simulink model "plant"  (R2026a)
settings: Solver=VariableStepAuto
undefined symbols (not defined in the file): pmsm
libraries: mcbplantlib x1, autolibpmsminterior x1
settings Model: Creator=probst  LastModifiedBy=probst

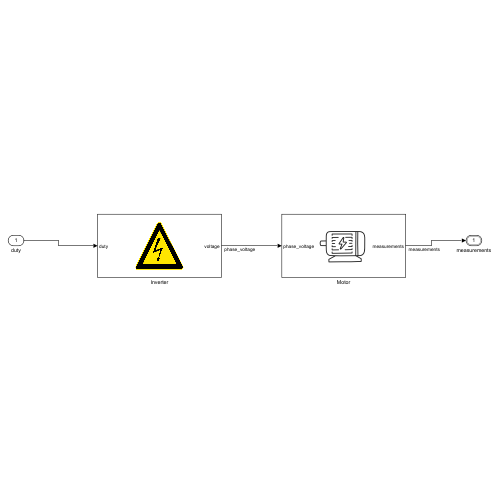
[thumbnail: Simulink's stored preview of the top-level diagram]
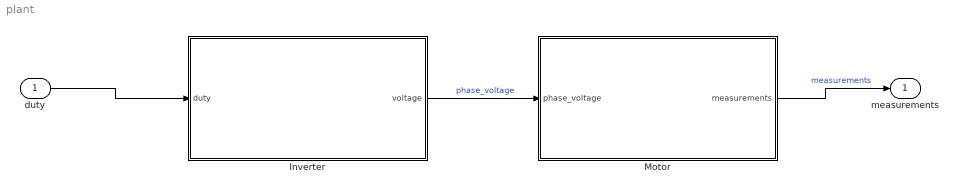
== system plant ==
  duty : Inport  OutDataTypeStr=double  PortDimensions=3
  Inverter : Subsystem
  Motor : Subsystem
  measurements : Outport  OutDataTypeStr=Bus: plant_measurement
  wires:
  duty/1 -> Inverter/1(duty)
  Inverter/1(voltage) -> Motor/1(phase_voltage)  "phase_voltage"
  Motor/1(measurements) -> measurements/1  "measurements"

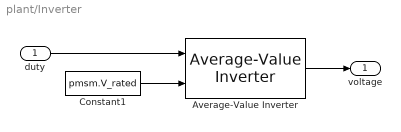
== system plant/Inverter ==
  duty : Inport
  Average-Value Inverter : mcbplantlib/Average-Value Inverter
      settings: LibrarySourceBlock=mcblib/Electrical Systems/Inverters/Average-Value Inverter
  Constant1 : Constant  Value=pmsm.V_rated
  voltage : Outport
  wires:
  Average-Value Inverter/1 -> voltage/1
  duty/1 -> Average-Value Inverter/1
  Constant1/1 -> Average-Value Inverter/2

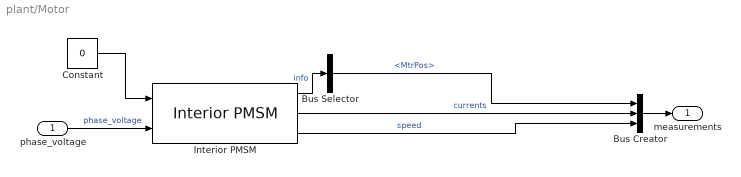
== system plant/Motor ==
  phase_voltage : Inport
  Bus Creator : BusCreator  Inputs=3  OutDataTypeStr=Bus: plant_measurement  NonVirtualBus=on
  Bus Selector : BusSelector  OutputSignals=MtrPos
  Constant : Constant  Value=0
  Interior PMSM : autolibpmsminterior/Interior PMSM  port_config=Torque  sim_type=Continuous  Ts=0.001  P=pmsm.P  Rs=pmsm.Rs  Ldq=pmsm.Ldq  KConstText=Permanent flux linkage constant (lambda_pm):  lambda_pm=pmsm.fl  Ke=pmsm.Ke  mechanical=pmsm.mechanical  idq0=[0 0]  theta_init=0  omega_init=0  KConst=pmsm.fl  lambda_pm_calc=pmsm.fl  Kt=0.07  RefBlkName='autolibpmsminterior/Interior PMSM'  aMode=5
      settings: LibrarySourceBlock=mcblib/Electrical Systems/Motors/Interior PMSM
  measurements : Outport  OutDataTypeStr=Bus: plant_measurement
  wires:
  Constant/1 -> Interior PMSM/1
  Bus Selector/1 -> Bus Creator/1  "<MtrPos>"
  Interior PMSM/2 -> Bus Creator/2  "currents"
  Interior PMSM/1 -> Bus Selector/1  "info"
  phase_voltage/1 -> Interior PMSM/2  "phase_voltage"
  Interior PMSM/3 -> Bus Creator/3  "speed"
  Bus Creator/1 -> measurements/1
